simulink model "IMU_board_example_Sensors_grouped"  (R2016a)
settings: Solver=ode1  StartTime=0.0  StopTime=inf  FixedStep=.0005  RelTol=1e-3
undefined symbols (not defined in the file or in its folder): deg, s
libraries: IMUboard_library x1, QB_pacer_lib x1, qbmove_library x1
settings Model: Creator=laurentio  LastModifiedBy=emanuele
settings DataIOCC: LimitDataPoints=on  SaveFormat=Array
settings DebuggingCC: UnderspecifiedInitializationDetection=Classic  MergeDetectMultiDrivingBlocksExec=none  SolverPrmCheckMsg=warning  AllowSymbolicDim=off  StateNameClashWarn=warning
settings HardwareCC: ProdBitPerPointer=32  ProdLargestAtomicFloat=None  ProdIntDivRoundTo=Undefined  ProdEndianess=Unspecified  ProdWordSize=32  ProdHWDeviceType=32-bit Generic
settings ModelReferenceCC: PropagateSignalLabelsOutOfModel=off
settings ConfigComp: CovModelRefEnable=Off  CovSFcnEnable=off

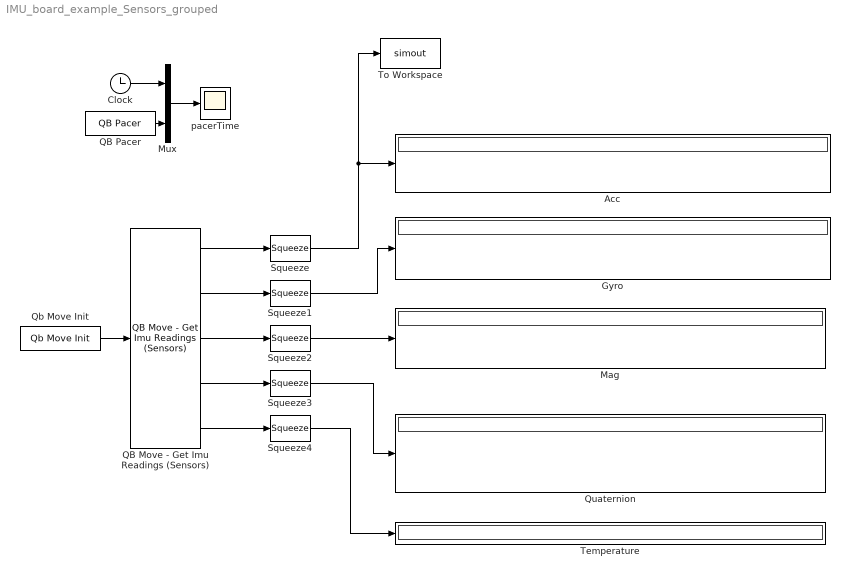
== system IMU_board_example_Sensors_grouped ==
  Acc : Display
  Clock : Clock
  Gyro : Display
  Mag : Display
  Mux : Mux  Inputs=2
  QB Move - Get Imu Readings (Sensors) : IMUboard_library/QB Move - Get Imu Readings (Sensors)  ID=1  N_IMU=5  DAISY_CHAINING=off  ACC_UNITY=G  GYRO_UNITY=deg/s  MAG_UNITY=uT
  QB Pacer : QB_pacer_lib/QB Pacer  simTimePerRealTime=1
  Qb Move Init : qbmove_library/Qb Move Init  NUMBER_OF_COM='COM2'  BAUD_RATE_COM=2000000
  Quaternion : Display
  Squeeze{,1..4} (5 alike) : Squeeze
  Temperature : Display
  To Workspace : ToWorkspace  VariableName=simout  SaveFormat=Timeseries  SampleTime=-1
  pacerTime : Scope
  wires:
  QB Pacer/1 -> Mux/2
  Clock/1 -> Mux/1
  Qb Move Init/1 -> QB Move - Get Imu Readings (Sensors)/1
  Mux/1 -> pacerTime/1
  QB Move - Get Imu Readings (Sensors)/1 -> Squeeze/1
  QB Move - Get Imu Readings (Sensors)/2 -> Squeeze1/1
  QB Move - Get Imu Readings (Sensors)/3 -> Squeeze2/1
  QB Move - Get Imu Readings (Sensors)/4 -> Squeeze3/1
  QB Move - Get Imu Readings (Sensors)/5 -> Squeeze4/1
  Squeeze/1 -> To Workspace/1, Acc/1
  Squeeze1/1 -> Gyro/1
  Squeeze2/1 -> Mag/1
  Squeeze3/1 -> Quaternion/1
  Squeeze4/1 -> Temperature/1
